simulink model "Rectifier"  (R2018a)
settings: Solver=VariableStepAuto  StartTime=0.0  StopTime=0.1  RelTol=1e-3
libraries: powerlib x11, powerlib_meascontrol x5
settings Model: Creator=Sadat Zubin Shah  LastModifiedBy=Sadat Zubin Shah

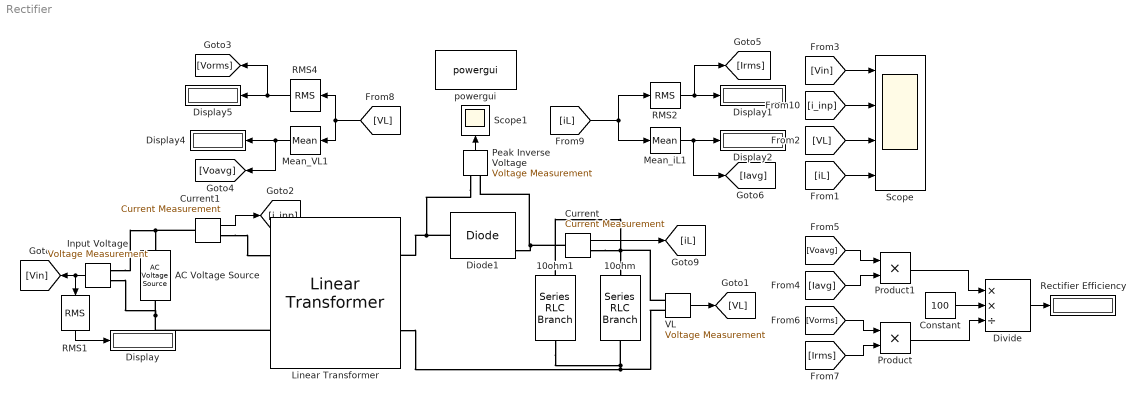
== system Rectifier ==
  10ohm : powerlib/Elements/Series RLC Branch  LConnTagsString=__new0  RConnTagsString=__new0  BranchType=R  Resistance=10  Inductance=1e-3  SetiL0=off  InitialCurrent=0  Capacitance=1e-6  Setx0=off  InitialVoltage=0  Measurements=None
  10ohm1 : powerlib/Elements/Series RLC Branch  LConnTagsString=__new0  RConnTagsString=__new0  BranchType=C  Resistance=10  Inductance=1e-3  SetiL0=off  InitialCurrent=0  Capacitance=1e-3  Setx0=off  InitialVoltage=0  Measurements=None
  AC Voltage Source : powerlib/Electrical Sources/AC Voltage Source  Amplitude=230*sqrt(2)  Phase=0  Frequency=50  SampleTime=0  Measurements=None  BusType=swing  Pref=10e3  Qref=0  Qmin=-inf  Qmax=+inf
  Constant : Constant  Value=100
  Current : powerlib/Measurements/Current Measurement  PhasorSimulation=off  OutputType=Complex  PSBequivalent=0
  Current1 : powerlib/Measurements/Current Measurement  PhasorSimulation=off  OutputType=Complex  PSBequivalent=0
  Diode1 : powerlib/Power Electronics/Diode  Ron=0.001  Lon=0  Vf=0.0  IC=0  UseSnubber=0  Rs=500  Cs=250e-9  Measurements=on
  Display{,1..2,4..5} (5 alike) : Display
  Divide : Product  Inputs=**/
  Input Voltage : powerlib/Measurements/Voltage Measurement  PhasorSimulation=off  OutputType=Complex  PSBequivalent=0
  Linear Transformer : powerlib/Elements/Linear Transformer  UNITS=SI  NominalPower=[1e3 50]  winding1=[230 0 0]  winding2=[6 0 0]  ThreeWindings=off  winding3=[3.15e+05 0.7938 0.084225]  RmLm=[500 500]  Measurements=None  DataType=on
  Mean_VL1 : powerlib_meascontrol/Measurements/Mean  Freq=50  Vinit=0  Ts=0
  Mean_iL1 : powerlib_meascontrol/Measurements/Mean  Freq=50  Vinit=0  Ts=0
  Peak Inverse Voltage : powerlib/Measurements/Voltage Measurement  PhasorSimulation=off  OutputType=Complex  PSBequivalent=0
  Product : Product
  Product1 : Product
  RMS1 : powerlib_meascontrol/Measurements/RMS  TrueRMS=on  Freq=50  RMSInit=0  Ts=0
  RMS2 : powerlib_meascontrol/Measurements/RMS  TrueRMS=on  Freq=50  RMSInit=0  Ts=0
  RMS4 : powerlib_meascontrol/Measurements/RMS  TrueRMS=on  Freq=50  RMSInit=0  Ts=0
  Rectifier Efficiency : Display
  Scope : Scope  NumInputPorts=4
  Scope1 : Scope
  VL : powerlib/Measurements/Voltage Measurement  PhasorSimulation=off  OutputType=Complex  PSBequivalent=0
  powergui : powerlib/powergui  Priority=1  SimulationMode=Discrete  SampleTime=50e-6  frequency=60  Iterations=50  frequencyindice=50  Pbase=100e6  ErrMax=1e-4  UnitsV=kV  UnitsW=MW  buscounter=0  FunctionMessages=off  echomessages=off  EnableUseOfTLC=off  CurrentSourceSwitches=off  DisableSnubberDevices=off  DisableRonSwitches=off  DisableVfSwitches=off  DisplayEquations=off  SolverType=Tustin/Backward Euler (TBE)  Interpol=off  ExternalGateDelay=off  methode=off  Ts=100  x0status=blocks  SPID=on  SwTol=0  HookPort=off  RestoreLinks=warning  ResistiveCurrentMeasurement=off  Frange=[0:2:500]  Ylog=off  Xlog=on  ShowGrid=off  save=off  variable=ZData  structure=0  ZoomFFT=off  StartTime=0.0  cycles=1  DisplayStyle=1  fundamental=60  FreqAxis=off  MaxFrequency=1000  frequencyindicesteady=1  RmsSteady=1  display=off
  wires:
  RMS1/1 -> Display/1
  Current/1 -> [iL]
  [Vin] -> Scope/1
  [VL] -> Scope/3
  [iL] -> Scope/4
  Peak Inverse Voltage/1 -> Scope1/1
  Product1/1 -> Divide/1
  Divide/1 -> Rectifier Efficiency/1
  VL/1 -> [VL]
  Constant/1 -> Divide/2
  [Voavg] -> Product1/1
  [Iavg] -> Product1/2
  [Irms] -> Product/2
  [Vorms] -> Product/1
  Product/1 -> Divide/3
  Input Voltage/1 -> [Vin], RMS1/1
  RMS4/1 -> Display5/1, [Vorms]
  [VL] -> RMS4/1, Mean_VL1/1
  Mean_VL1/1 -> Display4/1, [Voavg]
  Mean_iL1/1 -> Display2/1, [Iavg]
  [iL] -> RMS2/1, Mean_iL1/1
  RMS2/1 -> Display1/1, [Irms]
  Current1/1 -> [i_inp]
  [i_inp] -> Scope/2
  connections:
  Input Voltage/LConn1 -- Current1/LConn1 -- AC Voltage Source/RConn1
  Linear Transformer/LConn2 -- Input Voltage/LConn2 -- AC Voltage Source/LConn1
  Current/RConn1 -- 10ohm/LConn1 -- 10ohm1/LConn1 -- VL/LConn1
  Peak Inverse Voltage/LConn2 -- Diode1/LConn1 -- Linear Transformer/RConn1
  Current/LConn1 -- Peak Inverse Voltage/LConn1 -- Diode1/RConn1
  VL/LConn2 -- Linear Transformer/RConn2 -- 10ohm1/RConn1 -- 10ohm/RConn1
  Current1/RConn1 -- Linear Transformer/LConn1
